simulink model "SSA"  (R2020a)
settings: Solver=ode23s  StartTime=0.0  StopTime=2  MaxStep=1e-4  RelTol=1e-3
libraries: powerlib x16, re_lib x5, powerlib_meascontrol x1
settings Model: Creator=Mahesh Krishna  LastModifiedBy=vankurua
settings DataIOCC: ReturnWorkspaceOutputs=off
settings OptimizationCC: LifeSpan=inf
settings DebuggingCC: ArithmeticOperatorsInVariantConditions=warning
settings SFSimCC: SimUseLocalCustomCode=off  CustomCodeUndefinedFunction=UseInterfaceOnly
settings RTWCC: RTWUseLocalCustomCode=off
settings CodeAppCC: StateflowObjectComments=on
settings SimscapeCC: SimscapeNormalizeSystem=off

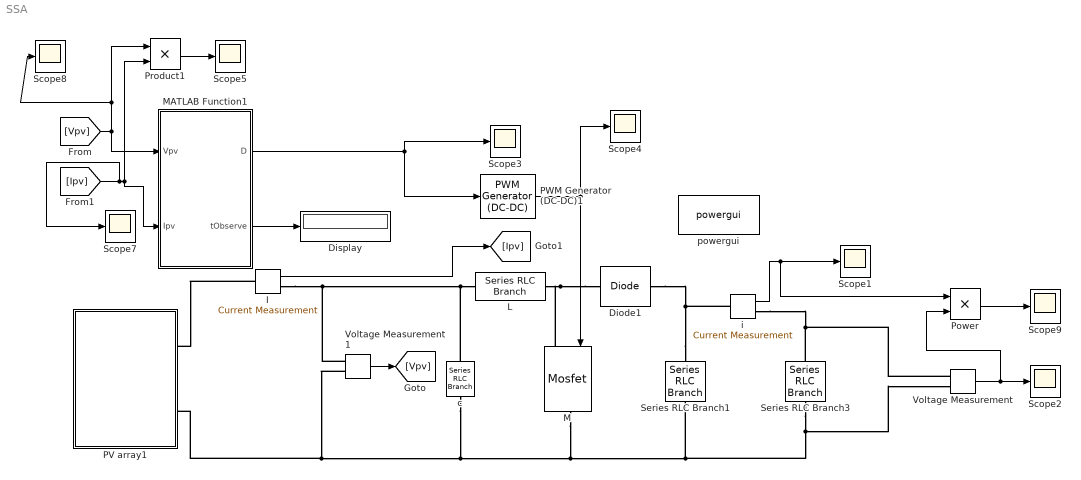
== system SSA ==
  Diode1 : powerlib/Power Electronics/Diode  Ron=1e-3  Lon=0  Vf=0  IC=0  UseSnubber=off  Rs=inf  Cs=inf  Measurements=off
  Display : Display
  I : powerlib/Measurements/Current Measurement  PhasorSimulation=off  OutputType=Magnitude  PSBequivalent=0
  L : powerlib/Elements/Series RLC Branch  LConnTagsString=__new0  RConnTagsString=__new0  BranchType=L  Resistance=1e-3  Inductance=5e-3  SetiL0=off  InitialCurrent=0  Capacitance=1e-6  Setx0=off  InitialVoltage=0  Measurements=None
  M : powerlib/Power Electronics/Mosfet  Ron=1e-3  Lon=0  Rd=1e-3  Vfd=0  IC=0  Rs=inf  Cs=inf  Measurements=off
  MATLAB Function1 : MATLAB Function  TreatAsAtomicUnit=on
  PV array1 : Subsystem
  PWM Generator (DC-DC)1 : powerlib_meascontrol/Pulse & Signal Generators/PWM Generator (DC-DC)  Fsw=20000  Ts=0
  Power : Product
  Product1 : Product
  Scope{1..5,7..9} (8 alike) : Scope
  Series RLC Branch1 : powerlib/Elements/Series RLC Branch  LConnTagsString=__new0  RConnTagsString=__new0  BranchType=C  Resistance=1e-4  Inductance=200e-6  SetiL0=off  InitialCurrent=0  Capacitance=22e-6  Setx0=off  InitialVoltage=40  Measurements=None
  Series RLC Branch3 : powerlib/Elements/Series RLC Branch  LConnTagsString=__new0  RConnTagsString=__new0  BranchType=R  Resistance=100  Inductance=200e-6  SetiL0=off  InitialCurrent=0  Capacitance=1000e-6  Setx0=off  InitialVoltage=40  Measurements=None
  Voltage Measurement : powerlib/Measurements/Voltage Measurement  PhasorSimulation=off  OutputType=Magnitude  PSBequivalent=0
  Voltage Measurement1 : powerlib/Measurements/Voltage Measurement  PhasorSimulation=off  OutputType=Magnitude  PSBequivalent=0
  c : powerlib/Elements/Series RLC Branch  LConnTagsString=__new0  RConnTagsString=__new0  BranchType=C  Resistance=1e-3  Inductance=250e-6  SetiL0=off  InitialCurrent=0  Capacitance=2.2e-6  Setx0=off  InitialVoltage=0  Measurements=None
  i : powerlib/Measurements/Current Measurement  PhasorSimulation=off  OutputType=Magnitude  PSBequivalent=0
  powergui : powerlib/powergui  Priority=1  SimulationMode=Continuous  SampleTime=50e-6  frequency=60  Iterations=50  frequencyindice=0  Pbase=100e6  ErrMax=1e-4  UnitsV=kV  UnitsW=MW  buscounter=0  FunctionMessages=off  echomessages=off  EnableUseOfTLC=off  CurrentSourceSwitches=off  DisableSnubberDevices=off  DisableRonSwitches=off  DisableVfSwitches=off  DisplayEquations=off  AutomaticDiscreteSolvers=off  SolverType=Tustin/Backward Euler (TBE)  Interpol=off  ExternalGateDelay=off  methode=off  Ts=100  x0status=blocks  SPID=on  SwTol=0  HookPort=off  NonlinearTolerance=1e-4  nMaxIteration=100  ContinueOnMaxIteration=off  RestoreLinks=warning  ResistiveCurrentMeasurement=off  Frange=[0:2:500]  Ylog=off  Xlog=on  ShowGrid=off  save=off  variable=ZData  structure=0  ZoomFFT=off  StartTime=0.0  cycles=1  DisplayStyle=1  fundamental=60  FreqAxis=off  MaxFrequency=1000  frequencyindicesteady=1  RmsSteady=1  display=off
  wires:
  I/1 -> [Ipv]
  [Ipv] -> Scope7/1, MATLAB Function1/2(Ipv), Product1/2
  Voltage Measurement/1 -> Power/2, Scope2/1
  PWM Generator (DC-DC)1/1 -> Scope4/1, M/1
  i/1 -> Power/1, Scope1/1
  Voltage Measurement1/1 -> [Vpv]
  [Vpv] -> MATLAB Function1/1(Vpv), Scope8/1, Product1/1
  Product1/1 -> Scope5/1
  Power/1 -> Scope9/1
  MATLAB Function1/1(D) -> Scope3/1, PWM Generator (DC-DC)1/1
  MATLAB Function1/2(tObserve) -> Display/1
  connections:
  i/RConn1 -- Series RLC Branch3/LConn1 -- Voltage Measurement/LConn1
  Series RLC Branch1/RConn1 -- Series RLC Branch3/RConn1 -- Voltage Measurement/LConn2 -- Voltage Measurement1/LConn2 -- PV array1/RConn2 -- c/RConn1 -- M/RConn1
  Series RLC Branch1/LConn1 -- Diode1/RConn1 -- i/LConn1
  I/LConn1 -- PV array1/RConn1
  Diode1/LConn1 -- M/LConn1 -- L/RConn1
  I/RConn1 -- Voltage Measurement1/LConn1 -- c/LConn1 -- L/LConn1

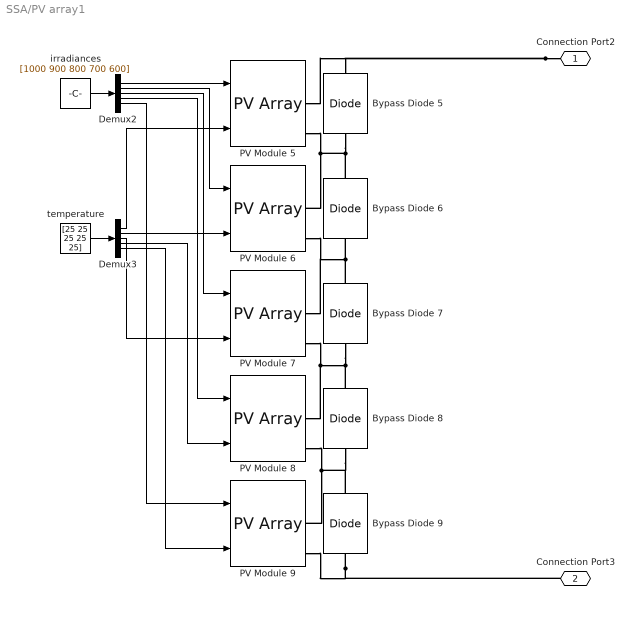
== system SSA/PV array1 ==
  Bypass Diode {5..9} (5 alike) : powerlib/Power Electronics/Diode  Ron=0.001  Lon=0  Vf=0.8  IC=0  UseSnubber=off  Rs=500  Cs=250e-9  Measurements=off
  Demux2 : Demux  Outputs=5
  Demux3 : Demux  Outputs=5
  PV Module 5 : re_lib/Solar/PV Array  Npar=1  Nser=1  PlotType=array @ 25 deg.C & specified irradiances  S_vec="[ 1000  500  100 ]"  Temp_C_vec="[ 45 25  ]"  ModuleName=1Soltech 1STH-215-P  PlotWhenSelected=off  Pm=213.15  Ncell=60  Voc=36.3  Isc=7.84  Vm=29  Im=7.35  beta_Voc_pc=-0.36099  alpha_Isc_pc=0.102  beta_Voc=-0.13104  alpha_Isc=0.007997  IL=7.8649  I0=2.9259e-10  nI=0.98117  Rsh=313.3991  Rs=0.39383  RobustModel=off  RobustCellTemperature=25  BAL=off  Tc=1e-6  Tfilter=5e-5
  PV Module {6..9} (4 alike) : re_lib/Solar/PV Array  Npar=1  Nser=1  PlotType=array @ 1000 W/m2 & specified temperatures  S_vec="[ 1000  500  100 ]"  Temp_C_vec="[ 45 25  ]"  ModuleName=1Soltech 1STH-215-P  PlotWhenSelected=off  Pm=213.15  Ncell=60  Voc=36.3  Isc=7.84  Vm=29  Im=7.35  beta_Voc_pc=-0.36099  alpha_Isc_pc=0.102  beta_Voc=-0.13104  alpha_Isc=0.007997  IL=7.8649  I0=2.9259e-10  nI=0.98117  Rsh=313.3991  Rs=0.39383  RobustModel=off  RobustCellTemperature=25  BAL=off  Tc=1e-6  Tfilter=5e-5
  irradiances : Constant  Value=[1000 900 800 700 600]
  temperature : Constant  Value=[25 25 25 25 25]
  Connection Port2 : PMIOPort  Side=Right
  Connection Port3 : PMIOPort  Port=2  Side=Right
  wires:
  Demux2/1 -> PV Module 5/1
  Demux3/4 -> PV Module 8/2
  Demux3/1 -> PV Module 5/2
  Demux3/3 -> PV Module 7/2
  Demux2/5 -> PV Module 9/1
  Demux2/4 -> PV Module 8/1
  Demux2/3 -> PV Module 7/1
  Demux3/5 -> PV Module 9/2
  irradiances/1 -> Demux2/1
  Demux2/2 -> PV Module 6/1
  temperature/1 -> Demux3/1
  Demux3/2 -> PV Module 6/2
  connections:
  Bypass Diode 6/RConn1 -- Bypass Diode 5/LConn1 -- PV Module 5/RConn2 -- PV Module 6/RConn1
  Connection Port2/RConn1 -- PV Module 5/RConn1 -- Bypass Diode 5/RConn1
  Bypass Diode 9/LConn1 -- Connection Port3/RConn1 -- PV Module 9/RConn2
  Bypass Diode 7/RConn1 -- Bypass Diode 6/LConn1 -- PV Module 7/RConn1 -- PV Module 6/RConn2
  PV Module 8/RConn2 -- PV Module 9/RConn1 -- Bypass Diode 8/LConn1 -- Bypass Diode 9/RConn1
  PV Module 7/RConn2 -- PV Module 8/RConn1 -- Bypass Diode 7/LConn1 -- Bypass Diode 8/RConn1

== matlab function SSA/MATLAB Function1 ==
  settings: updateMethod=DISCRETE  sampleTime=1e-4
  data: Vpv input; D output; Ipv input; tObserve output
function [D, tObserve] = SSA(Vpv,Ipv)
    N = 3; %粒子个数

    Xmin = 0; %粒子下限位置
    Xmax = 0.95; %粒子上限位置
    
    T = 20; %设最大迭代次数为T;
    persistent t; %设定当前迭代次数
    
    persistent P; %设P为种群
    persistent Fitness; %设Fitness为储存适应度信息的数组;
    
    persistent FoodPosition; %食物位置
    persistent FoodFitness; %适应度
    
    persistent dcurrent;
    persistent counter; %计数 用于稳定
    persistent u;
 
  
    
    if(isempty(t))
        t=1;
    end
    
    
    if(isempty(Fitness))
        Fitness = zeros(N,1);
    end
    
    if(isempty(P))
        P = zeros(N,1);
        step = (Xmax-Xmin)/N;
        for i = 1:N
            P(i) = Xmin+step*i;
        end
        
    end
    if(isempty(u))
        u=0;
    end
    if(isempty(dcurrent))
        dcurrent=0;
    end
    if(isempty(FoodPosition))
        FoodPosition=0;
    end
    if(isempty(FoodFitness))
        FoodFitness=0;
    end
    if(isempty(counter))
        counter=0;
    end
    

    tObserve = t;
    
    
    if(counter>=1 && counter<150)
        D=dcurrent;
        counter=counter+1;
        return;
    end
    
    counter=0;
    
    if(u>=1 && u<=N)
        Fitness(u) = Ipv*Vpv;
        if(Fitness(u)>=FoodFitness)
            FoodPosition = P(u);
            FoodFitness = Fitness(u);
        end
    end
    u = u+1;
    
    if(u>=1 && u<=N)
        D = P(u);
        dcurrent = D;
        counter = 1;
        return;
    end


   c1 = 2*exp(-(4*t/T)^2); %c1表示在开发和探索之间的平衡的值 越小 越偏向于开发，越大，越偏向于探索


    %更新salp粒子位置
    if(t>=T)
        w = 1;
    else
        w = t/T;
    end
    
    if round(w*N)<2
        LeaderCount = 1;
    else
        LeaderCount = round(w*N);
    end
    
    for i=1:N
        if i <=1  %其实我觉得这个探索粒子也可以做动态化处理
            c2 = rand();
            c3 = rand();
            if c3<0.5
                P(i)=FoodPosition+c1*((Xmax-Xmin)*c2+Xmin); 
            else
                P(i)=FoodPosition-c1*((Xmax-Xmin)*c2+Xmin);
            end
            % Update the position of the salp based on the second half of the swarm
        else
            point1 = P(i-1);
            point2 = P(i);
            
            P(i) = (point1+point2)/2;
        end
    end
    
    %如果超出边界了就取边界值
    for i = 1:N
        Tp = P(i)>Xmax; %超出上边界Tp = 0
        Tm = P(i)<Xmin; %超出下边界Tm = 0;
                     %或非  如果超出边界就取边界值，没有就是原来的    
                     %这里用了一个还算巧妙的算法 或非  如果超出边界就取边界值，没有就是原来的  
         P(i) = ( P(i) * (~(Tp+Tm)) )+Xmax*Tp+Xmin*Tm;
        
    end
    u=1;
    D = P(1);
    dcurrent = D;
    counter = 1;
    t=t+1; %更新t    
end

function dfinal=levyflight(dbest,d)
beta=3/2;
kcoeff=0.8;
sigmau=(gamma(1+beta)*sin(pi*beta/2)/(gamma((1+beta)/2)*beta*2^((beta-1)/2)))^(1/beta);
sigmav=1;
u=normrnd(0,(sigmau)^2);
v=normrnd(0,(sigmav)^2);
dup=d+(kcoeff*(abs(u)/((abs(v))^(1/beta)))*(dbest-d));


if(dup>1)
    dfinal=1;
elseif(dup<0)
    dfinal=0;
else
    dfinal=dup;
end
end
